simulink model "TRAMI_STEP_AT_vehicle_ver01_Jmaab_R2018b_Intg"  (R2018b)
settings: Solver=ode8  StartTime=0  StopTime=end_time  FixedStep=sampling_time  RelTol=1e-3
PreLoadFcn:
  | %init_setting;
values from neighbouring files (symbols this model uses):
  sampling_time = 0.0025    [METI_TRAMI_Thermal_ver01_Jmaab_PreLoad.m]
undefined symbols (not defined in the file or in its folder): ACC_D_Gain, ACC_I_Gain, ACC_P_Gain, ALT_CNT_ALT_OFF_RPM_HYS_rpm, ALT_CNT_ALT_ON_RPM_HYS_rpm, ALT_CNT_Alter_V_BASE_V, ALT_CNT_Alter_V_Kaisei_V, ALT_CNT_flag_disable_kaisei, ALT_CNT_V_Battely_Kudo_V, ALT_PNT_ALT_GDCurrent_A, ALT_PNT_ALT_GDVolt_V, ALT_PNT_Alter_limit_Current_V_table, ALT_PNT_Alter_limit_Current_V_table_x_rpm, ALT_PNT_Alter_trq_Nm_map, ALT_PNT_Alter_trq_Nm_map_x_rpm, ALT_PNT_Alter_trq_Nm_map_y_Current_A, ALT_PNT_Alter_trq_Nm_map_z_Volt_tgt_V, ALT_PNT_eta_pulley_alt, ALT_PNT_Gain_Alt_v_del, ALT_PNT_ratio_pulley_alt, ALT_PNT_Tau_Alternator_V_tgt_s, ALT_PNT_trq_alter_output_LL_Nm, BK_PNT_Pow_UL, BK_PNT_Tau_brake, Brk_LL, Brk_PGain, Brk_UL, BT_PNT_Lo_Capa_lo_batt_F, BT_PNT_Lo_ocv_SOC_lo_batt_OCV_V_table, BT_PNT_Lo_ocv_SOC_lo_batt_OCV_V_table_x_SOC, BT_PNT_Lo_R_lo_batt_ohm, BT_PNT_Lo_SOC_MAX_lo_batt, BT_PNT_Lo_SOC_MIN_lo_batt, BT_PNT_Lo_SOC_START_lo_batt, BT_PNT_Lo_V_start_ocv, Driver_Brake_Const1, Driver_Brake_Const3, Driver_Brake_Switch_Const2, Driver_Brk_sh, drivmode_ACC, drivmode_CONST, drivmode_GensokuKaisei, drivmode_GensokuRikko, drivmode_STOP, EL_PNT_R_bodyelec_lo_ohm, ENG_CNT_Accel_LL, ENG_CNT_Accel_UL, ENG_CNT_brak_idlestop, ENG_CNT_flag_idle_stop_exe, ENG_CNT_gain_p_per_isc, ENG_CNT_IdleSpeed_Const, ENG_CNT_omg_eng_fuelcut_rpm, ENG_CNT_per_isc_max, ENG_CNT_per_isc_min, ENG_CNT_per_throttle_fuelcut, ENG_CNT_per_throttle_isc_fb, ENG_CNT_Starter_timer_Const_s, ENG_CNT_Throttle_LL, ENG_CNT_Throttle_UL, ENG_CNT_V_car_idlestop_kmph ... (+29)
libraries: METI_Lib_vehicle_model x18, simulink x4, AZAPA_Lib_vehicle_model x1
(part 3 of 3)

== system TRAMI_STEP_AT_vehicle_ver01_Jmaab_R2018b_Intg/Vehicle/CNT/ENG_CNT/ENG_Cntrl/Set_Idle_Stop ==
  note: ○アイドリングストップ制御
      | 　停車時＋ブレーキを踏んでいるとき、アイドリングストップ
  v_vehicle : Inport
  per_brake : Inport  Port=2
  Constant : Constant  Value=ENG_CNT_V_car_idlestop_kmph
  Constant1 : Constant  Value=ENG_CNT_brak_idlestop
  Constant2 : Constant  Value=ENG_CNT_flag_idle_stop_exe
  Logical Operator : Logic  Inputs=3  AllPortsSameDT=off  OutDataTypeStr=boolean
  Relational Operator : RelationalOperator  Operator=<  OutDataTypeStr=boolean  RndMeth=Nearest
  Relational Operator1 : RelationalOperator  OutDataTypeStr=boolean  RndMeth=Nearest
  flag_IdleStop : Outport
  wires:
  Relational Operator/1 -> Logical Operator/2
  Logical Operator/1 -> flag_IdleStop/1
  v_vehicle/1 -> Relational Operator/1
  per_brake/1 -> Relational Operator1/1
  Constant/1 -> Relational Operator/2
  Constant1/1 -> Relational Operator1/2
  Relational Operator1/1 -> Logical Operator/3
  Constant2/1 -> Logical Operator/1

== system TRAMI_STEP_AT_vehicle_ver01_Jmaab_R2018b_Intg/Vehicle/CNT/ENG_CNT/ENG_Cntrl/Starter ==
  note: サンプリング時間
  note: 時間リセット
  note: アイドリングフラグがON→OFFに
      | 切り替わり時スターターON開始
  note: スタータ開始時間
  note: スタータ開始時間から
      | ある時間超えたらOFF
  note: アイドリングフラグがON→OFFに切り替わり時スターターON開始.ある時間を超えたらOFF
  flag_idlestop : Inport
  n_eng_rpm : Inport  Port=2
  Constant2 : Constant  Value=ENG_CNT_Starter_timer_Const_s
  Constant4 : Constant  Value=sampling_time
  Constant5 : Constant  Value=0
  Constant6 : Constant  Value=OFF
  Constant7 : Constant  Value=ON
  IdleSpeed : Constant  Value=ENG_CNT_IdleSpeed_Const/2
  Logical Operator : Logic  Inputs=3  AllPortsSameDT=off  OutDataTypeStr=boolean
  Logical Operator1 : Logic  Operator=NOT  AllPortsSameDT=off  OutDataTypeStr=boolean
  Memory : Memory  InitialCondition=1000
  Memory1 : Memory  InheritSampleTime=on
  Relational Operator1 : RelationalOperator  Operator=<=  OutDataTypeStr=boolean  RndMeth=Nearest
  Relational Operator2 : RelationalOperator  Operator=<  OutDataTypeStr=boolean  RndMeth=Nearest
  Sum5 : Sum  Inputs=|++
  Switch3 : Switch  Criteria=u2 > Threshold  Threshold=0.5
  Switch4 : Switch  Criteria=u2 > Threshold  Threshold=0.5
  flag_ON_Starter : Outport
  wires:
  Switch4/1 -> flag_ON_Starter/1
  Memory/1 -> Sum5/2
  Constant4/1 -> Sum5/1
  Constant5/1 -> Switch3/1
  Sum5/1 -> Switch3/3
  Switch3/1 -> Relational Operator1/1, Memory/1
  Memory1/1 -> Logical Operator/2
  Logical Operator1/1 -> Logical Operator/1
  flag_idlestop/1 -> Memory1/1, Logical Operator1/1
  Logical Operator/1 -> Switch3/2
  Constant2/1 -> Relational Operator1/2
  Relational Operator1/1 -> Switch4/2
  Constant7/1 -> Switch4/1
  Constant6/1 -> Switch4/3
  n_eng_rpm/1 -> Relational Operator2/1
  IdleSpeed/1 -> Relational Operator2/2
  Relational Operator2/1 -> Logical Operator/3

== system TRAMI_STEP_AT_vehicle_ver01_Jmaab_R2018b_Intg/Vehicle/CNT/TM_CNT/TM_CNT/T_PT_TH_K ==
  From Workspace1 : FromWorkspace  VariableName=T_PT_TH_K  SampleTime=0  OutputAfterFinalValue=Holding final value
  Sum2 : Sum  Inputs=|++
  ℃⇒K : Constant  Value=273.15
  Out1 : Outport
  wires:
  From Workspace1/1 -> Sum2/1
  ℃⇒K/1 -> Sum2/2
  Sum2/1 -> Out1/1

== system TRAMI_STEP_AT_vehicle_ver01_Jmaab_R2018b_Intg/Vehicle/ENG_PNT/ENG_Plant/Cal_FuelComsunption/Not_cal1 ==
  In1 : Inport
  Constant : Constant  Value=0
  Constant1 : Constant
  Switch : Switch  Criteria=u2 > Threshold  Threshold=0.5
  Out1 : Outport
  wires:
  Constant1/1 -> Switch/3
  Constant/1 -> Switch/1
  Switch/1 -> Out1/1
  In1/1 -> Switch/2

== system TRAMI_STEP_AT_vehicle_ver01_Jmaab_R2018b_Intg/Vehicle/ENG_PNT/ENG_Plant/Cal_FuelComsunption/Not_cal2 ==
  In1 : Inport
  Constant : Constant  Value=0
  Constant1 : Constant
  Switch : Switch  Criteria=u2 > Threshold  Threshold=0.5
  Out1 : Outport
  wires:
  In1/1 -> Switch/2
  Switch/1 -> Out1/1
  Constant/1 -> Switch/1
  Constant1/1 -> Switch/3

== system TRAMI_STEP_AT_vehicle_ver01_Jmaab_R2018b_Intg/Vehicle/ENG_PNT/ENG_Plant/Cal_trq_ENG_jiku/Not_cal ==
  In1 : Inport
  Constant : Constant  Value=0
  Constant1 : Constant
  Switch : Switch  Criteria=u2 > Threshold  Threshold=0.5
  Out1 : Outport
  wires:
  In1/1 -> Switch/2
  Switch/1 -> Out1/1
  Constant/1 -> Switch/1
  Constant1/1 -> Switch/3

== system TRAMI_STEP_AT_vehicle_ver01_Jmaab_R2018b_Intg/Vehicle/ENG_PNT/ENG_Plant/Cal_trq_ENG_jiku/Not_cal1 ==
  In1 : Inport
  Constant : Constant  Value=0
  Constant1 : Constant
  Switch : Switch  Criteria=u2 > Threshold  Threshold=0.5
  Out1 : Outport
  wires:
  Constant1/1 -> Switch/3
  Constant/1 -> Switch/1
  Switch/1 -> Out1/1
  In1/1 -> Switch/2

== system TRAMI_STEP_AT_vehicle_ver01_Jmaab_R2018b_Intg/Vehicle/CNT/ENG_CNT/ENG_Cntrl/Caliculate_Idle_Speed/Subsystem ==
  del_omg_engine : Inport
  flag_idle_fb : Inport  Port=2
  Gain : Gain  Gain=ENG_CNT_gain_p_per_isc
  Logical Operator1 : Logic  Operator=NOT  AllPortsSameDT=off  OutDataTypeStr=boolean
  Memory : Memory  InitialCondition=4
  Saturation : Saturate  UpperLimit=ENG_CNT_per_isc_max  LowerLimit=ENG_CNT_per_isc_min
  Switch : Switch  Criteria=u2 > Threshold  Threshold=0.5
  per_isc_[%] : Outport
  wires:
  Switch/1 -> Saturation/1
  flag_idle_fb/1 -> Logical Operator1/1
  Gain/1 -> Switch/3
  Memory/1 -> Switch/1
  Saturation/1 -> per_isc_[%]/1, Memory/1
  del_omg_engine/1 -> Gain/1
  Logical Operator1/1 -> Switch/2

== system TRAMI_STEP_AT_vehicle_ver01_Jmaab_R2018b_Intg/Vehicle/CNT/ENG_CNT/ENG_Cntrl/Caliculate_Idle_Speed/Subsystem1 ==
  note: アイドル回転数時のFB
  omg_tgt_idle : Inport
  n_eng_rpm : Inport  Port=2
  per_throttle_base : Inport  Port=3
  flag_Lockup : Inport  Port=4
  flag_IdleStop : Inport  Port=5
  Logical Operator : Logic  Operator=OR  AllPortsSameDT=off  OutDataTypeStr=boolean
  Logical Operator1 : Logic  Operator=NOT  AllPortsSameDT=off  OutDataTypeStr=boolean
  Logical Operator2 : Logic  Inputs=3  AllPortsSameDT=off  OutDataTypeStr=boolean
  Logical Operator3 : Logic  Operator=NOT  AllPortsSameDT=off  OutDataTypeStr=boolean
  Logical Operator4 : Logic  Operator=NOT  AllPortsSameDT=off  OutDataTypeStr=boolean
  Logical Operator5 : Logic  AllPortsSameDT=off  OutDataTypeStr=boolean
  Relational Operator : RelationalOperator  Operator=<  OutDataTypeStr=boolean  RndMeth=Nearest
  Relational Operator2 : RelationalOperator  Operator=>  OutDataTypeStr=boolean  RndMeth=Nearest
  per_throttle_isc_fb : Constant  Value=ENG_CNT_per_throttle_isc_fb
  flag_idle_fb : Outport
  wires:
  per_throttle_base/1 -> Relational Operator/1
  per_throttle_isc_fb/1 -> Relational Operator/2
  Relational Operator2/1 -> Logical Operator2/1
  Relational Operator/1 -> Logical Operator1/1, Logical Operator5/1
  Logical Operator1/1 -> Logical Operator2/2
  Logical Operator5/1 -> Logical Operator/2
  flag_Lockup/1 -> Logical Operator3/1
  Logical Operator3/1 -> Logical Operator2/3
  Logical Operator2/1 -> Logical Operator/1
  omg_tgt_idle/1 -> Relational Operator2/1
  n_eng_rpm/1 -> Relational Operator2/2
  flag_IdleStop/1 -> Logical Operator4/1
  Logical Operator4/1 -> Logical Operator5/2
  Logical Operator/1 -> flag_idle_fb/1
